simulink model "IA331_lab10_1"  (R2023b)
settings: Solver=VariableStepAuto  StartTime=0.0  StopTime=50.0  RelTol=1e-3
model workspace (MAT data in the model file):
  lambda = 5
  max_prio = 10
  p_drop = 0.5
  service_time = 2
  u = 6
undefined symbols (not defined in the file): m, n
settings Model: Creator=jjake  LastModifiedBy=jjake

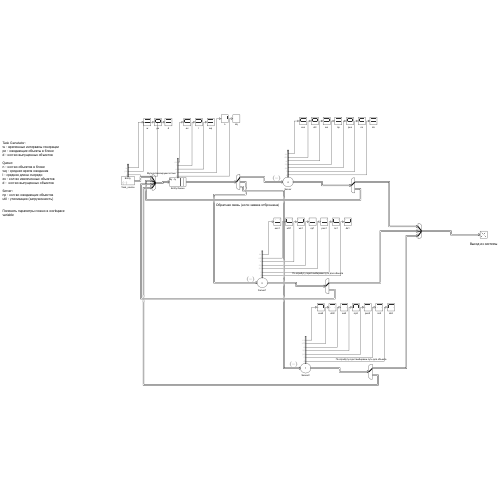
[thumbnail: Simulink's stored preview of the top-level diagram]
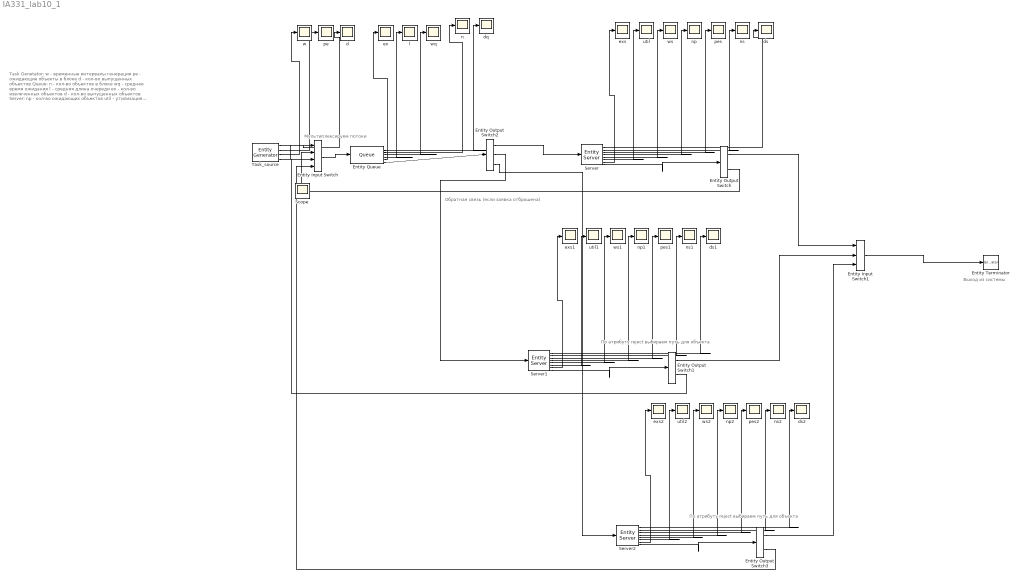
== system IA331_lab10_1 ==
  note: Мультиплексируем потоки
  note: Выход из системы
  note: Обратная связь (если заявка отброшена)
  note: Task Genetator:
      | w - временные интервалы генерации
      | pe - ожидающие объекты в блоке
      | d - кол-во выпущенных объектов
      |
      | Queue:
      | n - кол-во объектов в блоке
      | wq - среднее время ожидания
      | l - средняя длина очереди
      | ex - кол-во извлеченных объектов
      | d - кол-во выпущенных объектов
      |
      | Server:
      | np - кол-во ожидающих объектов
      | util - утилизация (загруженность)
      |
      | Поменять параметры можно в workspace
      | variable
  note: По атрибуту reject выбираем путь для объекта
  note: По атрибуту reject выбираем путь для объекта
  Entity Input Switch : EntityInputSwitch  InputPortMessageModes=m,m,m,m  OutputPortMessageModes=m  NumberInputPorts=4
      settings: InputPortMap=u1,u2,u3,u4
  Entity Input Switch1 : EntityInputSwitch  InputPortMessageModes=m,m,m  OutputPortMessageModes=m  NumberInputPorts=3
      settings: InputPortMap=u1,u2,u3
  Entity Output Switch : EntityOutputSwitch  InputPortMessageModes=m  OutputPortMessageModes=m,m  SwitchingCriterion=From attribute  SwitchAttributeName=reject
  Entity Output Switch1 : EntityOutputSwitch  InputPortMessageModes=m  OutputPortMessageModes=m,m  SwitchingCriterion=From attribute  SwitchAttributeName=reject
  Entity Output Switch2 : EntityOutputSwitch  InputPortMessageModes=m  OutputPortMessageModes=m,m,m  NumberOutputPorts=3  SwitchingCriterion=Round robin  SwitchAttributeName=Attribute1
      settings: OutputPortMap=o0,o1,o2
  Entity Output Switch3 : EntityOutputSwitch  InputPortMessageModes=m  OutputPortMessageModes=m,m  SwitchingCriterion=From attribute  SwitchAttributeName=reject
  Entity Queue : Queue  InputPortMessageModes=m  OutputPortMessageModes=n,n,n,n,n,m  Capacity=100  QueueType=Priority  PrioritySource=priority  NumberEntitiesDeparted=on  NumEntitiesExtracted=on  NumberEntitiesInBlock=on  AverageWait=on  AverageQueueLength=on
      settings: OutputPortMap=o0,o1,o2,o3,o7,o5
  Entity Terminator : EntityTerminator  InputPortMessageModes=m
  Server : EntityServer  InputPortMessageModes=m  OutputPortMessageModes=n,n,n,n,n,n,n,m  Capacity=4  ServiceTimeSource=MATLAB action  ServiceTimeAction=dt = exprnd(1/100);  EntryAction=|  SortingAttributeName=priority  NumberEntitiesDeparted=on  NumberEntitiesInBlock=on  PendingEntityPresentInBlock=on  NumberEntitiesPending=on  AverageWait=on  Utilization=on  NumEntitiesExtracted=on
      | persistent rngInit;
      | if isempty(rngInit)
      |     seed = 12345;
      |     rng(seed);
      |     rngInit = true;
      | end
      | 
      | if rand < p_drop
      |     entity.reject = 1;
      | else
      |     entity.reject = 2;
      | end
      settings: OutputPortMap=o0,o1,o2,o3,o4,o5,o12,o9
  Server1 : EntityServer  InputPortMessageModes=m  OutputPortMessageModes=n,n,n,n,n,n,n,m  Capacity=3  ServiceTimeSource=MATLAB action  ServiceTimeAction=dt = exprnd(1/u);  EntryAction=|  SortingAttributeName=priority  NumberEntitiesDeparted=on  NumberEntitiesInBlock=on  PendingEntityPresentInBlock=on  NumberEntitiesPending=on  AverageWait=on  Utilization=on  NumEntitiesExtracted=on
      | persistent rngInit;
      | if isempty(rngInit)
      |     seed = 12345;
      |     rng(seed);
      |     rngInit = true;
      | end
      | 
      | if rand < p_drop
      |     entity.reject = 1;
      | else
      |     entity.reject = 2;
      | end
      settings: OutputPortMap=o0,o1,o2,o3,o4,o5,o12,o9
  Server2 : EntityServer  InputPortMessageModes=m  OutputPortMessageModes=n,n,n,n,n,n,n,m  Capacity=1  ServiceTimeSource=MATLAB action  ServiceTimeAction=dt = exprnd(1/u);  EntryAction=|  SortingAttributeName=priority  NumberEntitiesDeparted=on  NumberEntitiesInBlock=on  PendingEntityPresentInBlock=on  NumberEntitiesPending=on  AverageWait=on  Utilization=on  NumEntitiesExtracted=on
      | persistent rngInit;
      | if isempty(rngInit)
      |     seed = 12345;
      |     rng(seed);
      |     rngInit = true;
      | end
      | 
      | if rand < p_drop
      |     entity.reject = 1;
      | else
      |     entity.reject = 2;
      | end
      settings: OutputPortMap=o0,o1,o2,o3,o4,o5,o12,o9
  Task_source : EntityGenerator  OutputPortMessageModes=n,n,n,m  TimeSource=MATLAB action  Period=1/1000  IntergenerationTimeAction=dt = exprnd(1/lambda);  GenerateAction=|  AttributeName=priority|reject  AttributeInitialValue=1|1  NumberEntitiesDeparted=on  PendingEntityInBlock=on  AverageIntergenerationTime=on  EntityType=Structured  EntityTypeName=Entity  EntityPriority=1
      | persistent rngInit id;
      | if isempty(rngInit)
      |     seed = 12345;
      |     rng(seed);
      |     rngInit = true;
      |     id = 0;
      | end
      | 
      | % Pattern: Uniform distribution
      | % m: Minimum, M: Maximum
      | m = 0; M = max_prio;
      | Task_source.priority = m + (M - m) * rand;
      settings: OutputPortMap=o0,o1,o2,o3
  d : Scope
  dq : Scope
  ds : Scope
  ds1 : Scope
  ds2 : Scope
  ex : Scope
  exs : Scope
  exs1 : Scope
  exs2 : Scope
  l : Scope
  n : Scope
  np : Scope
  np1 : Scope
  np2 : Scope
  ns : Scope
  ns1 : Scope
  ns2 : Scope
  pe : Scope
  pes : Scope
  pes1 : Scope
  pes2 : Scope
  util : Scope
  util1 : Scope
  util2 : Scope
  w : Scope
  wq : Scope
  ws : Scope
  ws1 : Scope
  ws2 : Scope
  Scope : Scope
  wires:
  Task_source/3 -> w/1
  Task_source/2 -> pe/1
  Task_source/1 -> d/1
  Server/7 -> exs/1
  Server/6 -> util/1
  Server/5 -> ws/1
  Server/4 -> np/1
  Server/3 -> pes/1
  Server/2 -> ns/1
  Server/1 -> ds/1
  Server/8 -> Entity Output Switch/1
  Entity Queue/5 -> ex/1
  Entity Queue/4 -> l/1
  Entity Queue/3 -> wq/1
  Entity Queue/2 -> n/1
  Entity Queue/1 -> dq/1
  Task_source/4 -> Entity Input Switch/1
  Entity Output Switch/2 -> Entity Input Switch/2
  Entity Input Switch/1 -> Entity Queue/1
  Server1/2 -> ns1/1
  Server1/4 -> np1/1
  Server1/1 -> ds1/1
  Server1/3 -> pes1/1
  Server1/6 -> util1/1
  Server1/8 -> Entity Output Switch1/1
  Server1/7 -> exs1/1
  Server1/5 -> ws1/1
  Entity Queue/6 -> Entity Output Switch2/1
  Entity Output Switch2/2 -> Server1/1
  Entity Output Switch/1 -> Entity Input Switch1/1
  Entity Output Switch1/1 -> Entity Input Switch1/2
  Server2/2 -> ns2/1
  Server2/4 -> np2/1
  Server2/1 -> ds2/1
  Server2/3 -> pes2/1
  Server2/6 -> util2/1
  Server2/8 -> Entity Output Switch3/1
  Server2/7 -> exs2/1
  Server2/5 -> ws2/1
  Entity Output Switch3/1 -> Entity Input Switch1/3
  Entity Output Switch2/3 -> Server2/1
  Entity Output Switch1/2 -> Entity Input Switch/3
  Entity Output Switch3/2 -> Entity Input Switch/4
  Entity Input Switch1/1 -> Entity Terminator/1
  Entity Output Switch2/1 -> Server/1
